simulink model "UnWaterChannelProbeTestSymmetry"  (Simulink 7.7)
settings: Solver=ode4  StartTime=0  StopTime=0.1  FixedStep=0.0001  RelTol=1e-3
undefined symbols (not defined in the file or in its folder): madnipcim
libraries: xpcnilib x1, dspsrcs4 x1, xpclib x1
settings Model: Creator=mvetsch  LastModifiedBy=newton  BufferReuse=off
settings DataIOCC: LimitDataPoints=off  SaveState=on  SignalLoggingName=logsOut
settings OptimizationCC: BlockReduction=off  BooleanDataType=off  OptimizeBlockIOStorage=off  BufferReuse=off  ExpressionFolding=off  LocalBlockOutputs=off  InitFltsAndDblsToZero=on
settings DebuggingCC: SaveWithParameterizedLinksMsg=none  CheckExecutionContextPreStartOutputMsg=on  CheckExecutionContextRuntimeOutputMsg=on  SignalResolutionControl=TryResolveAllWithWarning  SolverPrmCheckMsg=none  MultiTaskDSMMsg=warning  MultiTaskCondExecSysMsg=none  FcnCallInpInsideContextMsg=Enable All  StrictBusMsg=None
settings HardwareCC: ProdIntDivRoundTo=Zero  ProdEndianess=LittleEndian  ProdHWDeviceType=Generic->32-bit x86 compatible
settings RTWCC: SystemTargetFile=xpctarget.tlc  TemplateMakefile=xpc_default_tmf  Description=xPC Target  ProcessScript=xpctarget_make_rtw_hook  IncludeERTFirstTime=on  RTWCompilerOptimization=On
settings xpcTargetCC: TargetFcnLib=ansi_tfl_tmw.mat  TargetFunctionLibrary=XPC_BLAS  FunctionExecutionProfile=off  CodeExecutionProfiling=off  ERTCodeCoverageTool=None  ParMdlRefBuildCompliant=on  CombineSignalStateStructs=off  PortableWordSizes=off  xPCTaskExecutionProfile=off  xPCRL32EventNumber=5000  xPCLoadParamSetFile=off  xPCConcurrentTasks=off  xPCEnableSFAnimation=off

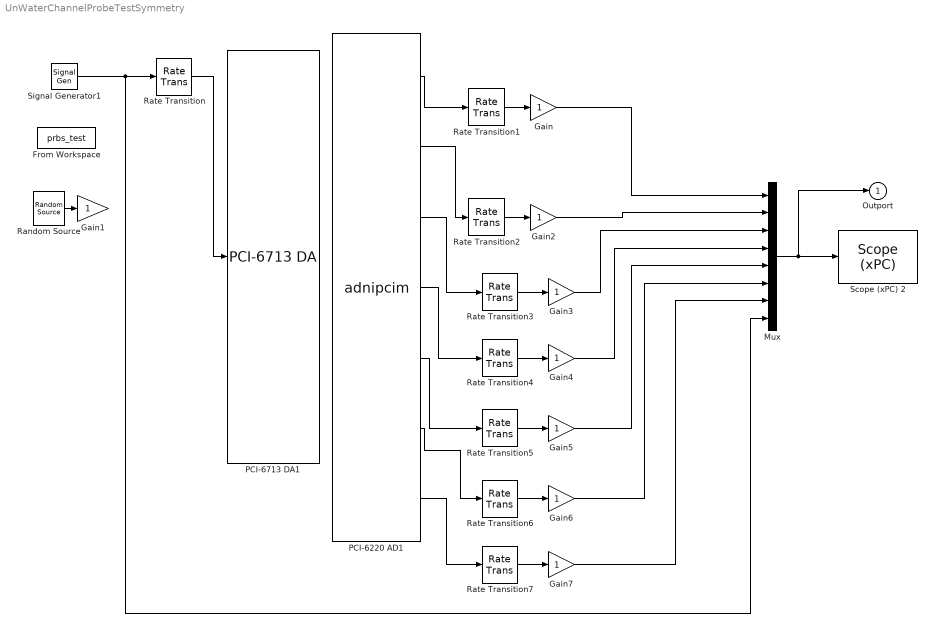
== system UnWaterChannelProbeTestSymmetry ==
  From Workspace : FromWorkspace  VariableName=prbs_test  SampleTime=1e-4  Interpolate=off  OutputAfterFinalValue=Setting to zero
  Gain{,1..7} (8 alike) : Gain
  Mux : Mux  Inputs=8
  PCI-6220 AD1 : S-Function  AncestorBlock=xpcnilib/A//D/M Series/PCI-6221 AD  InitFcn=madnipcim(1);  FunctionName=adnipcim  Parameters="channel, range, coupling, scantime, sampletime, slot,  boardType"  SFunctionModules=xpcionim  EnableBusSupport=off  mask(adnipci6221){channel=[1,2,3,4,5,6,7], range=[10], coupling=[0], scantime=5e-6, sampletime=1e-4, slot=-1}
      mask prompts: channel "Channel vector (1-16):"; range "Range vector (in the set [10, 5, 1, 0.2]):"; coupling "Input coupling vector (0: RSE, 1: NRSE, 2: DIFF):"; scantime "Scan Interval:"; sampletime "Sample time:"; slot "PCI slot (-1: autosearch):"
      mask help:
      | PCI-6221
      | National Instruments
      | Analog Input
      mask init:
      | boardType=20;
      | [maskdisplay, range, coupling, scantime] = madnipcim(2,channel, range, coupling, scantime, boardType);
      | set_param( gcb, 'MaskDisplay', maskdisplay );
      mask Help: eval('xpcdoc(''NationalInstruments_PCI-6221_AD'')');
      mask Display: disp('PCI-6220\nNational Instr.\nAnalog Input'); port_label('output', 1, '1'); port_label('output', 2, '2'); port_label('output', 3, '3'); port_label('output', 4, '4'); port_label('output', 5, '5'); port_label('output', 6, '6'); port_label('output', 7, '7');
  PCI-6713 DA1 : xpcnilib/D//A/PCI-6713 DA  channel=[1]  reset=[0]  initval=[0]  sampletime=1e-4  pcislot=-1
  Random Source : dspsrcs4/Random Source  SrcType=Uniform  NormMethod=Ziggurat  CltLength=12  MinVal=0  MaxVal=4  MeanVal=0  VarVal=1  RepMode=Not repeatable  rawSeed=1  IsInherit=off  SampMode=Continuous  SampTime=2e-4  SampFrame=1  DataType=Double  OutComplex=Real
  Rate Transition{,1..7} (8 alike) : RateTransition
  Scope (xPC) 2 : xpclib/Misc./Scope (xPC)   SystemSampleTime=-1  scopeno=4  scopetype=Target  autostart=on  viewmode=Graphical redraw  formatstr='%15.6f'  grid=on  ylimits=[0,0]  nosamples=100  noprepostsamples=0  interleave=1  triggermode=FreeRun  triggersignal=1  triggerlevel=0.0  triggerslope=Either  triggerscope=1  triggersample=0  filename=data.dat  mode=Lazy  writesize=512  autorestart=off  dynamicfilemode=off  maxwritefilesize=512*1024^2
  Signal Generator1 : SignalGenerator  WaveForm=square  Amplitude=10  Frequency=500
  Outport : Outport  InitialOutput=0
  wires:
  Rate Transition/1 -> PCI-6713 DA1/1
  PCI-6220 AD1/1 -> Rate Transition1/1
  Mux/1 -> Scope (xPC) 2/1, Outport/1
  Rate Transition1/1 -> Gain/1
  Random Source/1 -> Gain1/1
  Rate Transition2/1 -> Gain2/1
  PCI-6220 AD1/2 -> Rate Transition2/1
  Gain/1 -> Mux/1
  Gain2/1 -> Mux/2
  Rate Transition3/1 -> Gain3/1
  Gain3/1 -> Mux/3
  PCI-6220 AD1/3 -> Rate Transition3/1
  Rate Transition4/1 -> Gain4/1
  Rate Transition5/1 -> Gain5/1
  Rate Transition6/1 -> Gain6/1
  Gain4/1 -> Mux/4
  Gain5/1 -> Mux/5
  Gain6/1 -> Mux/6
  PCI-6220 AD1/4 -> Rate Transition4/1
  PCI-6220 AD1/5 -> Rate Transition5/1
  PCI-6220 AD1/6 -> Rate Transition6/1
  Signal Generator1/1 -> Rate Transition/1, Mux/8
  Rate Transition7/1 -> Gain7/1
  PCI-6220 AD1/7 -> Rate Transition7/1
  Gain7/1 -> Mux/7
